simulink model "PaperSim"  (R2022b)
settings: Solver=VariableStepAuto  StartTime=0.0  StopTime=10.0  RelTol=1e-3
settings Model: Creator=bob  LastModifiedBy=bob

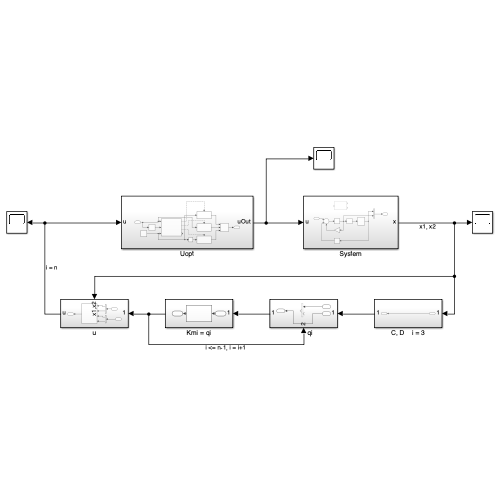
[thumbnail: Simulink's stored preview of the top-level diagram]
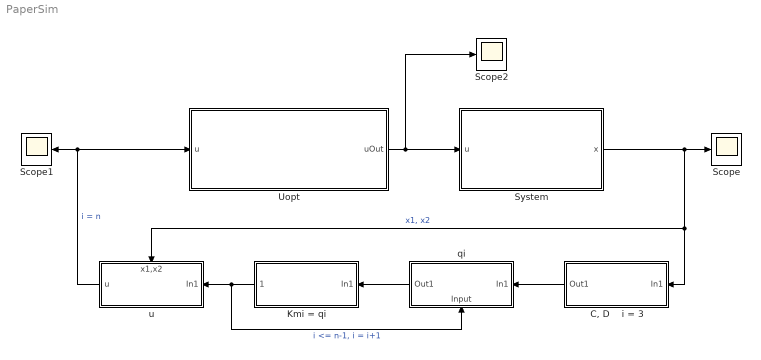
== system PaperSim ==
  "       qi" : Subsystem
      settings: PortSchema="{\"entries\":[{\"content\":{\"sides\":[{\"content\":{\"connectorIds\":[\"In1\"]},\"type\":\"ConnectorPlacement.EquallySpacedRectSide\",\"uuid\":\"a4180728-2693-404c-a392-844bb374b3ea\"},{\"content\":{\"connectorIds\":[\"Out1\"],\"side\":\"RIGHT\"},\"type\":\"ConnectorPlacement.EquallySpacedRectSide\",\"uuid\":\"543e197c-f9c3-4796-a178-018829468a5a\"},{\"content\":{\"connectorIds\":[],\"side\":\"TOP\"},\"type\":\"ConnectorPlacement.EquallySpacedRectSide\",\"uuid\":\"55e0f144-1543-48e8-a919-2318b9024530\"},{\"content\":{\"connectorIds\":[\"In2\"],\"side\":\"BOTTOM\"},\"type\":\"ConnectorPlacement.EquallySpacedRectSide\",\"uuid\":\"2d0b9248-44fb-437c-8189-235a787e0259\"}]},\"type\":\"ConnectorPlacement.EquallySpacedConnector\",\"uuid\":\"7f1c7ca5-0360-40d7-b631-2a4b3db23b13\"}],\"packageUris\":[\"http://schema.mathworks.com/mf0/Connector/R2020b\"],\"version\":\"1.0\"}"
  "C, D    i = 3" : Subsystem
  Kmi = qi : Subsystem
  Scope : Scope
  Scope1 : Scope
  Scope2 : Scope
  System : Subsystem
  Uopt : Subsystem
  u : Subsystem
      settings: PortSchema="{\"entries\":[{\"content\":{\"sides\":[{\"content\":{\"connectorIds\":[\"In1\"]},\"type\":\"ConnectorPlacement.EquallySpacedRectSide\",\"uuid\":\"a4180728-2693-404c-a392-844bb374b3ea\"},{\"content\":{\"connectorIds\":[\"Out1\"],\"side\":\"RIGHT\"},\"type\":\"ConnectorPlacement.EquallySpacedRectSide\",\"uuid\":\"543e197c-f9c3-4796-a178-018829468a5a\"},{\"content\":{\"connectorIds\":[\"In2\"],\"side\":\"TOP\"},\"type\":\"ConnectorPlacement.EquallySpacedRectSide\",\"uuid\":\"55e0f144-1543-48e8-a919-2318b9024530\"}]},\"type\":\"ConnectorPlacement.EquallySpacedConnector\",\"uuid\":\"7f1c7ca5-0360-40d7-b631-2a4b3db23b13\"}],\"packageUris\":[\"http://schema.mathworks.com/mf0/Connector/R2020b\"],\"version\":\"1.0\"}"
  wires:
  u/1(u) -> Scope1/1, Uopt/1(u)  "i = n"
  Kmi = qi/1(" ") -> "       qi"/2(Input), u/1(In1)  "i <= n-1, i = i+1"
  System/1(x) -> Scope/1, u/2(x1,x2), "C, D    i = 3"/1(In1)  "x1, x2"
  "C, D    i = 3"/1(Out1) -> "       qi"/1(In1)
  "       qi"/1(Out1) -> Kmi = qi/1(In1)
  Uopt/1(uOut) -> Scope2/1, System/1(u)

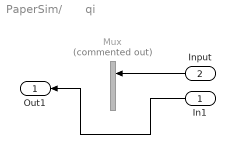
== system PaperSim/       qi ==
  In1 : Inport
  Input : Inport  Port=2
  Mux : Mux  Commented=on  Inputs=2
  Out1 : Outport
  wires:
  Input/1 -> Mux/1
  In1/1 -> Out1/1

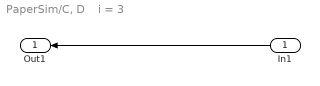
== system PaperSim/C, D    i = 3 ==
  In1 : Inport
  Out1 : Outport
  wires:
  In1/1 -> Out1/1

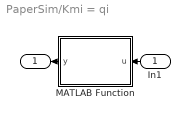
== system PaperSim/Kmi = qi ==
  In1 : Inport
  MATLAB Function : MATLAB Function  TreatAsAtomicUnit=on
  " " : Outport
  wires:
  In1/1 -> MATLAB Function/1(u)
  MATLAB Function/1(y) -> " "/1

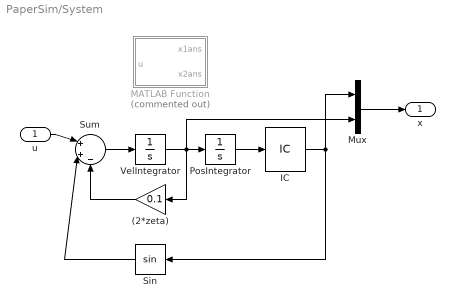
== system PaperSim/System ==
  u : Inport
  (2*zeta) : Gain  Gain=0.1
  IC : InitialCondition
  MATLAB Function : MATLAB Function  Commented=on  TreatAsAtomicUnit=on
  Mux : Mux  Inputs=2
  PosIntegrator : Integrator
  Sin : Trigonometry
  Sum : Sum  Inputs=|++-
  VelIntegrator : Integrator
  x : Outport
  wires:
  Mux/1 -> x/1
  u/1 -> Sum/1
  PosIntegrator/1 -> IC/1
  Sin/1 -> Sum/2
  VelIntegrator/1 -> PosIntegrator/1, Mux/2, (2*zeta)/1
  Sum/1 -> VelIntegrator/1
  (2*zeta)/1 -> Sum/3
  IC/1 -> Sin/1, Mux/1

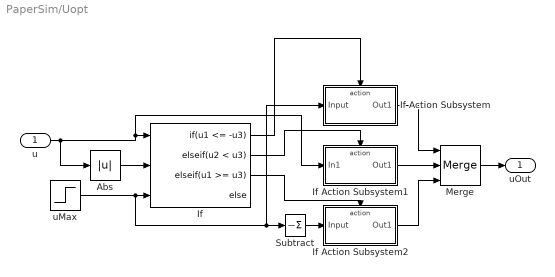
== system PaperSim/Uopt ==
  u : Inport
  Abs : Abs  SaturateOnIntegerOverflow=off
  If : If  NumInputs=3  IfExpression=u1 <= -u3  ElseIfExpressions=u2 < u3, u1 >= u3
  If Action Subsystem : Subsystem  TreatAsAtomicUnit=on
  If Action Subsystem1 : Subsystem  TreatAsAtomicUnit=on
  If Action Subsystem2 : Subsystem  TreatAsAtomicUnit=on
  Merge : Merge  Inputs=3
  Subtract : Sum  Inputs=-
  uMax : Step  Time=0  SampleTime=0
  uOut : Outport
  wires:
  u/1 -> If Action Subsystem1/1(In1), If/1, Abs/1
  Abs/1 -> If/2
  If/1 -> If Action Subsystem/Action
  If/2 -> If Action Subsystem1/Action
  If/3 -> If Action Subsystem2/Action
  Subtract/1 -> If Action Subsystem2/1(Input)
  Merge/1 -> uOut/1
  If Action Subsystem1/1(Out1) -> Merge/2
  If Action Subsystem/1(Out1) -> Merge/1
  If Action Subsystem2/1(Out1) -> Merge/3
  uMax/1 -> If Action Subsystem/1(Input), Subtract/1, If/3

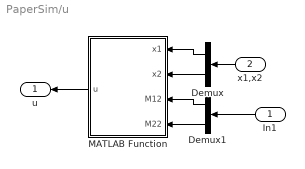
== system PaperSim/u ==
  In1 : Inport
  x1,x2 : Inport  Port=2
  Demux : Demux  Outputs=2
  Demux1 : Demux  Outputs=2
  MATLAB Function : MATLAB Function  TreatAsAtomicUnit=on
  u : Outport
  wires:
  MATLAB Function/1(u) -> u/1
  x1,x2/1 -> Demux/1
  Demux/1 -> MATLAB Function/1(x1)
  Demux/2 -> MATLAB Function/2(x2)
  In1/1 -> Demux1/1
  Demux1/1 -> MATLAB Function/3(M12)
  Demux1/2 -> MATLAB Function/4(M22)

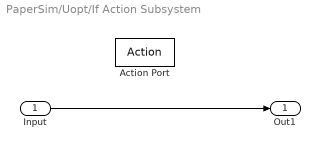
== system PaperSim/Uopt/If Action Subsystem ==
  Input : Inport
  Action Port : ActionPort  ActionPortLabel=if(u1 <= -u3)
  Out1 : Outport
  wires:
  Input/1 -> Out1/1

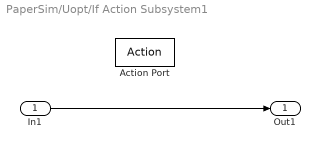
== system PaperSim/Uopt/If Action Subsystem1 ==
  In1 : Inport
  Action Port : ActionPort  ActionPortLabel=elseif(u2 < u3)
  Out1 : Outport
  wires:
  In1/1 -> Out1/1

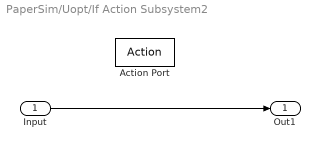
== system PaperSim/Uopt/If Action Subsystem2 ==
  Input : Inport
  Action Port : ActionPort  ActionPortLabel=elseif( u1 >= u3)
  Out1 : Outport
  wires:
  Input/1 -> Out1/1

== matlab function PaperSim/u/MATLAB Function ==
  data: u output; x1 input; x2 input; M12 input; M22 input
function u = fcn(x1,x2, M12, M22)

function beta = bOfx(x)

beta = sin(x)/x;

end

realM12 = 1;
realM22 = 1;
zeta = 0.08471;

a1 = realM22^2 + 2*zeta;

a2 = 1/(realM12^2) - (1/(realM22*2 + 2*zeta)^2);

u = -0.5*((2*(realM12^2)*x1 + 2*(realM22^2)*x2) + exp(1)*(2*bOfx(x1)*x1 + 2*(bOfx(x1)/a1)*x2)) ...
    + (exp(2))*(((bOfx(x1)^2)/(realM12^2))*x1 + (((bOfx(x1)^2)/a1)*a2*x2));

end

== matlab function PaperSim/System/MATLAB Function ==
  data: u input; x1ans output; x2ans output
function [x1ans,x2ans]= fcn(u)

syms x1 x2

ode1 = diff(x1) == x2;
ode2 = diff(x2) == sin(x1) - (2 * zeta * x2) + u;
odes = [ode1; ode2];

[x1ans, x2ans] = dsolve(odes);

== matlab function PaperSim/Kmi = qi/MATLAB Function ==
  data: u input; y output
function y = fcn(u)

y = u;
